simulink model "modeloPert"  (R2024b)
settings: Solver=VariableStepAuto  StartTime=0.0  StopTime=10.0  RelTol=1e-3
undefined symbols (not defined in the file): pert, step_value, Ts
settings Model: Creator=estel  LastModifiedBy=estel

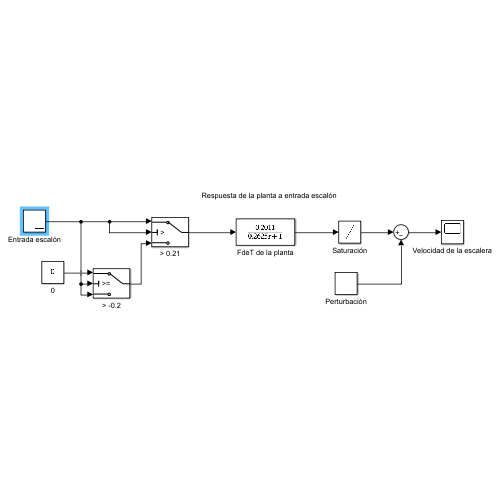
[thumbnail: Simulink's stored preview of the top-level diagram]
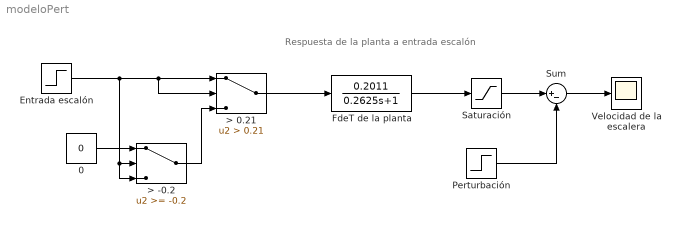
== system modeloPert ==
  note: Respuesta de la planta a entrada escalón
  0 : Constant  Value=0
  > -0.2 : Switch  Threshold=-0.2  SaturateOnIntegerOverflow=off  InputSameDT=off
  > 0.21 : Switch  Criteria=u2 > Threshold  Threshold=0.21  SaturateOnIntegerOverflow=off  InputSameDT=off
  Entrada escalón : Step  Time=0  After=step_value  SampleTime=Ts
  FdeT de la planta : TransferFcn  Numerator=0.2011  Denominator=[0.2625 1]
  Perturbación : Step  Time=2.5  After=pert  SampleTime=0
  Saturación : Saturate  UpperLimit=2.1098  LowerLimit=-2.1123
  Sum : Sum  Inputs=|+-
  Velocidad de la escalera : Scope
  wires:
  FdeT de la planta/1 -> Saturación/1
  Saturación/1 -> Sum/1
  Perturbación/1 -> Sum/2
  Sum/1 -> Velocidad de la escalera/1
  > -0.2/1 -> > 0.21/3
  0/1 -> > -0.2/1
  Entrada escalón/1 -> > -0.2/2, > -0.2/3, > 0.21/2, > 0.21/1
  > 0.21/1 -> FdeT de la planta/1
